simulink model "cruise_ctrl_17"  (R2017a)
settings: Solver=FixedStepAuto  StartTime=0.0  StopTime=60  FixedStep=0.01  MaxStep=0.1  RelTol=1e-3  EnableMultiTasking=on
PreLoadFcn:
  | m = 1000;
  | alpha = [40, 25, 16, 12, 10];
  | Tm = 190;
  | wm = 420;
  | beta = 0.4;
  | Cr = 0.01;
  | rho = 1.3;
  | Cd = 0.32;
  | A = 2.4;
  | g = 9.8;
  | theta = 0;
  | gear = 3;
libraries: simulink x2
settings Model: Creator=Cole Lepine  LastModifiedBy=nikhil
settings DataIOCC: LimitDataPoints=on  SaveFormat=Array
settings OptimizationCC: ExpressionDepthLimit=2147483647  InitFltsAndDblsToZero=on  LifeSpan=inf
settings DebuggingCC: UnderspecifiedInitializationDetection=Classic  MergeDetectMultiDrivingBlocksExec=none  SolverPrmCheckMsg=warning  FcnCallInpInsideContextMsg=warning  StateNameClashWarn=warning  SFUnexpectedBacktrackingDiag=warning  SFNoUnconditionalDefaultTransitionDiag=warning  SFExecutionAtInitializationDiag=none
settings HardwareCC: ProdBitPerPointer=32  ProdBitPerSizeT=32  ProdBitPerPtrDiffT=32  ProdLargestAtomicFloat=None  ProdIntDivRoundTo=Undefined  ProdEndianess=Unspecified  ProdWordSize=32  ProdHWDeviceType=32-bit Generic
settings ModelReferenceCC: PropagateSignalLabelsOutOfModel=off
settings GRTTargetCC: TargetLangStandard=C89/C90 (ANSI)  CombineOutputUpdateFcns=off  GRTInterface=on
settings ConfigComp: CovMetricSettings=dw  CovHtmlReporting=on  CovSaveCumulativeToWorkspaceVar=on  CovSaveSingleToWorkspaceVar=on  CovExternalEMLEnable=off

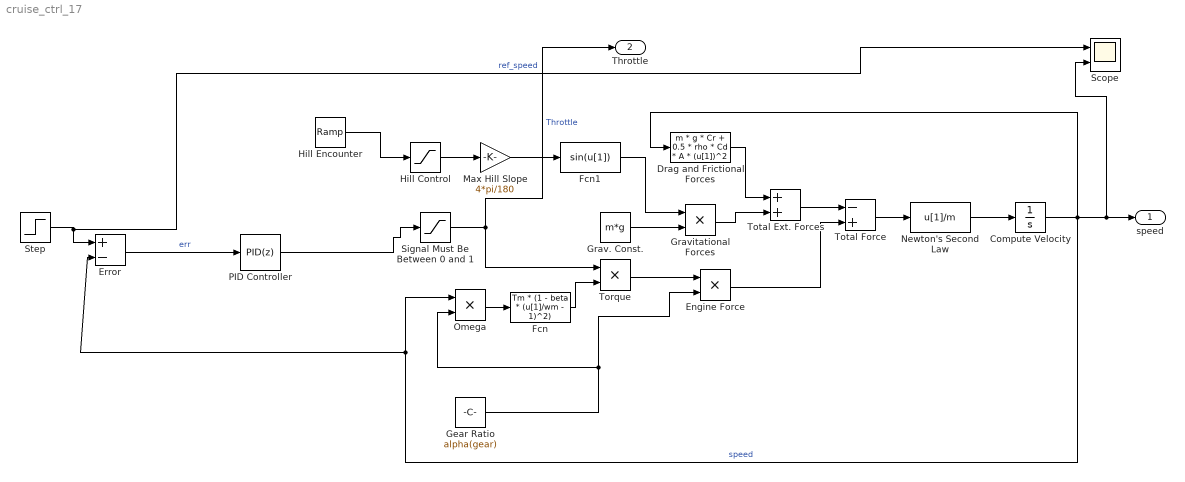
== system cruise_ctrl_17 ==
  Compute Velocity : Integrator  InitialCondition=20
  Drag and Frictional Forces : Fcn  Expr=m * g * Cr + 0.5 * rho * Cd * A * (u[1])^2
  Engine Force : Product  Inputs=**
  Error : Sum  Inputs=+-
  Fcn : Fcn  Expr=Tm * (1 - beta * (u[1]/wm - 1)^2)
  Fcn1 : Fcn
  Gear Ratio : Constant  Value=alpha(gear)
  Grav. Const. : Constant  Value=m*g
  Gravitational Forces : Product  RndMeth=Zero
  Hill Control : Saturate  UpperLimit=1  LowerLimit=0
  Hill Encounter : simulink/Sources/Ramp  slope=1  start=60  X0=0
  Max Hill Slope : Gain  Gain=4*pi/180
  Newton's Second Law : Fcn  Expr=u[1]/m
  Omega : Product  RndMeth=Zero
  PID Controller : simulink/Continuous/PID Controller  Controller=PID  TimeDomain=Discrete-time  SampleTime=-1  IntegratorMethod=Forward Euler  FilterMethod=Forward Euler  Form=Parallel  UseFilter=off  ControllerParametersSource=internal  P=1  I=5  D=20  N=100  InitialConditionSource=internal  InitialConditionForIntegrator=0  InitialConditionForFilter=0  ExternalReset=none  LimitOutput=off  UpperSaturationLimit=inf  LowerSaturationLimit=-inf  LinearizeAsGain=on  AntiWindupMode=none  Kb=1  TrackingMode=off  Kt=1  PParamMin=[]  PParamMax=[]  IParamMin=[]  IParamMax=[]  DParamMin=[]  DParamMax=[]  NParamMin=[]  NParamMax=[]  KbParamMin=[]  KbParamMax=[]  KtParamMin=[]  KtParamMax=[]  POutMin=[]  POutMax=[]  IOutMin=[]  IOutMax=[]  DOutMin=[]  DOutMax=[]  NOutMin=[]  NOutMax=[]  KbOutMin=[]  KbOutMax=[]  KtOutMin=[]  KtOutMax=[]  IntegratorOutMin=[]  IntegratorOutMax=[]  FilterOutMin=[]  FilterOutMax=[]  SumOutMin=[]  SumOutMax=[]  SumI1OutMin=[]  SumI1OutMax=[]  SumI2OutMin=[]  SumI2OutMax=[]  SumI3OutMin=[]  SumI3OutMax=[]  SumDOutMin=[]  SumDOutMax=[]  SaturationOutMin=[]  SaturationOutMax=[]  IntegratorContinuousStateAttributes=''  IntegratorStateMustResolveToSignalObject=off  IntegratorRTWStateStorageClass=Auto  FilterContinuousStateAttributes=''  FilterStateMustResolveToSignalObject=off  FilterRTWStateStorageClass=Auto  DifferentiatorICPrevScaledInput=0  DifferentiatorOutMin=[]  DifferentiatorOutMax=[]  InitialConditionSetting=Output
  Scope : Scope  NumInputPorts=2
  Signal Must Be Between 0 and 1 : Saturate  UpperLimit=1  LowerLimit=0
  Step : Step  Time=0  After=20  SampleTime=0
  Torque : Product  RndMeth=Zero
  Total Ext. Forces : Sum
  Total Force : Sum  Inputs=-+
  speed : Outport
  Throttle : Outport  Port=2
  wires:
  Engine Force/1 -> Total Force/2
  Total Force/1 -> Newton's Second Law/1
  Newton's Second Law/1 -> Compute Velocity/1
  Compute Velocity/1 -> Scope/2, speed/1, Drag and Frictional Forces/1, Omega/1, Error/2  "speed"
  Omega/1 -> Fcn/1
  Torque/1 -> Engine Force/1
  Fcn/1 -> Torque/2
  Signal Must Be Between 0 and 1/1 -> Throttle/1, Torque/1  "Throttle"
  Step/1 -> Scope/1, Error/1  "ref_speed"
  PID Controller/1 -> Signal Must Be Between 0 and 1/1
  Total Ext. Forces/1 -> Total Force/1
  Drag and Frictional Forces/1 -> Total Ext. Forces/1
  Gravitational Forces/1 -> Total Ext. Forces/2
  Fcn1/1 -> Gravitational Forces/1
  Max Hill Slope/1 -> Fcn1/1
  Grav. Const./1 -> Gravitational Forces/2
  Hill Control/1 -> Max Hill Slope/1
  Hill Encounter/1 -> Hill Control/1
  Error/1 -> PID Controller/1  "err"
  Gear Ratio/1 -> Engine Force/2, Omega/2
